simulink model "ProyectoFinalLA"  (R2023a)
settings: Solver=ode15s  StartTime=0  StopTime=30  MaxStep=1e-3  RelTol=1e-3
settings Model: Creator=piqui  LastModifiedBy=piqui
settings DataIOCC: ReturnWorkspaceOutputs=off  TimeSaveName=t
settings DebuggingCC: AlgebraicLoopMsg=none  ArtificialAlgebraicLoopMsg=none  MaxConsecutiveZCsMsg=none  ModelReferenceExtraNoncontSigs=none  OperatingPointInterfaceChecksumMismatchMsg=none

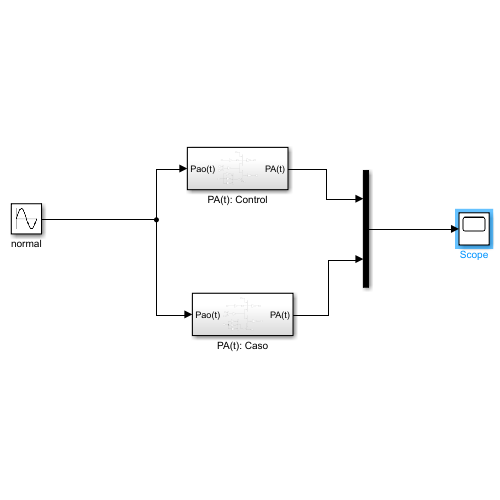
[thumbnail: Simulink's stored preview of the top-level diagram]
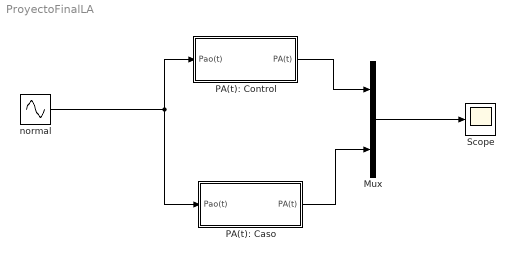
== system ProyectoFinalLA ==
  Mux : Mux  Inputs=2
  PA(t): Caso : Subsystem
  PA(t): Control : Subsystem
  Scope : Scope
  normal : Sin  Frequency=pi/2  SampleTime=0
  wires:
  normal/1 -> PA(t): Caso/1(Pao(t)), PA(t): Control/1(Pao(t))
  Mux/1 -> Scope/1
  PA(t): Control/1(PA(t)) -> Mux/1
  PA(t): Caso/1(PA(t)) -> Mux/2

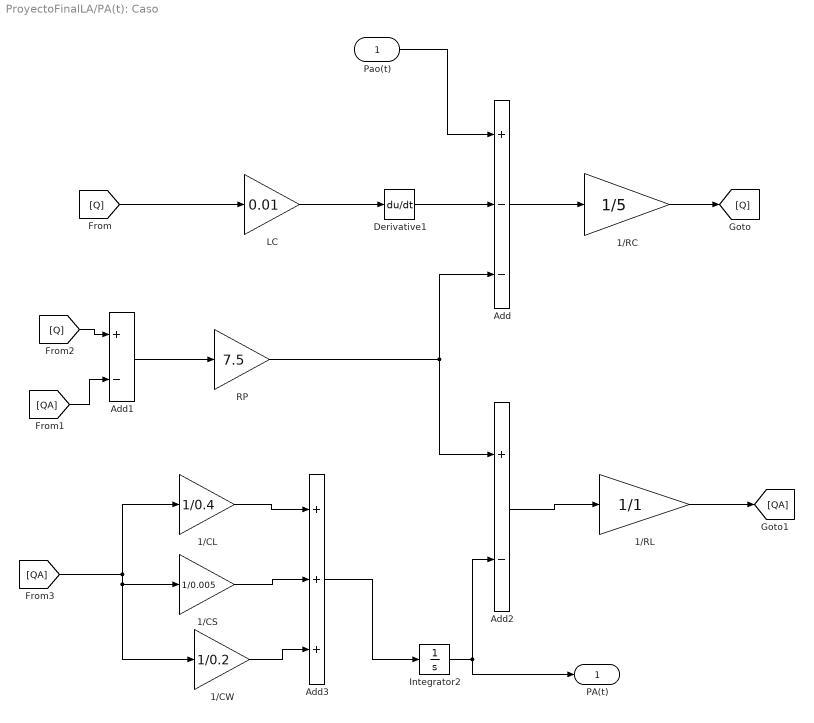
== system ProyectoFinalLA/PA(t): Caso ==
  Pao(t) : Inport
  1/CL : Gain  Gain=1/0.4
  1/CS : Gain  Gain=1/0.005
  1/CW : Gain  Gain=1/0.2
  1/RC : Gain  Gain=1/5
  1/RL : Gain  Gain=1/1
  Add : Sum  Inputs=+--
  Add1 : Sum  Inputs=+-
  Add2 : Sum  Inputs=+-
  Add3 : Sum  Inputs=+++
  Derivative1 : Derivative
  Integrator2 : Integrator
  LC : Gain  Gain=0.01
  RP : Gain  Gain=7.5
  PA(t) : Outport
  wires:
  1/CS/1 -> Add3/2
  Integrator2/1 -> Add2/2, PA(t)/1
  Add3/1 -> Integrator2/1
  Add2/1 -> 1/RL/1
  1/RC/1 -> [Q]
  1/CW/1 -> Add3/3
  Add1/1 -> RP/1
  1/CL/1 -> Add3/1
  [QA] -> 1/CS/1, 1/CW/1, 1/CL/1
  Derivative1/1 -> Add/2
  [Q] -> LC/1
  Pao(t)/1 -> Add/1
  RP/1 -> Add/3, Add2/1
  [QA] -> Add1/2
  LC/1 -> Derivative1/1
  [Q] -> Add1/1
  Add/1 -> 1/RC/1
  1/RL/1 -> [QA]

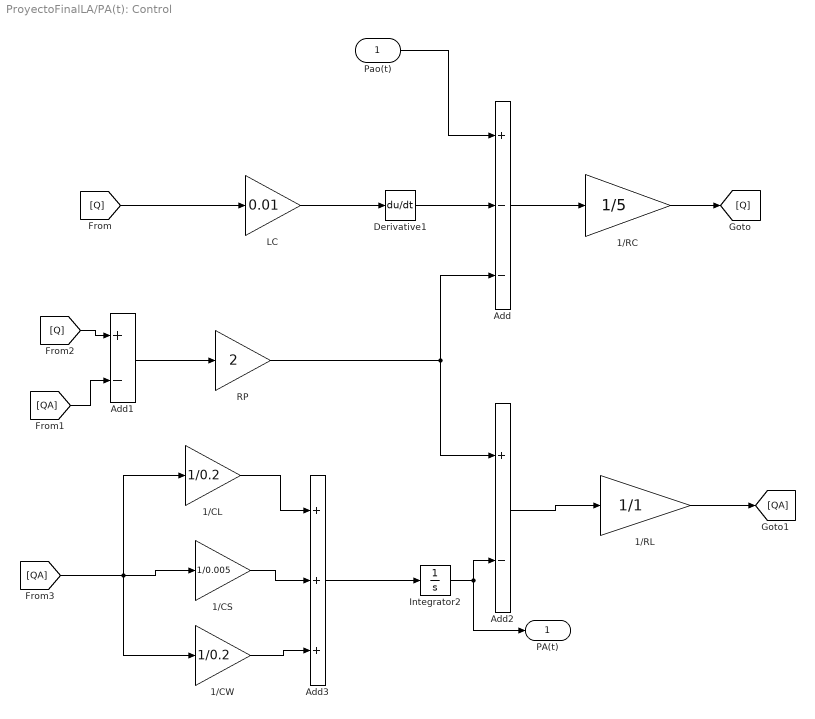
== system ProyectoFinalLA/PA(t): Control ==
  Pao(t) : Inport
  1/CL : Gain  Gain=1/0.2
  1/CS : Gain  Gain=1/0.005
  1/CW : Gain  Gain=1/0.2
  1/RC : Gain  Gain=1/5
  1/RL : Gain  Gain=1/1
  Add : Sum  Inputs=+--
  Add1 : Sum  Inputs=+-
  Add2 : Sum  Inputs=+-
  Add3 : Sum  Inputs=+++
  Derivative1 : Derivative
  Integrator2 : Integrator
  LC : Gain  Gain=0.01
  RP : Gain  Gain=2
  PA(t) : Outport
  wires:
  1/CW/1 -> Add3/3
  Integrator2/1 -> PA(t)/1, Add2/2
  1/CS/1 -> Add3/2
  RP/1 -> Add/3, Add2/1
  Derivative1/1 -> Add/2
  Add2/1 -> 1/RL/1
  Add/1 -> 1/RC/1
  [QA] -> 1/CW/1, 1/CS/1, 1/CL/1
  [QA] -> Add1/2
  Add3/1 -> Integrator2/1
  [Q] -> LC/1
  1/RL/1 -> [QA]
  1/CL/1 -> Add3/1
  Add1/1 -> RP/1
  LC/1 -> Derivative1/1
  1/RC/1 -> [Q]
  Pao(t)/1 -> Add/1
  [Q] -> Add1/1
